simulink model "NEWTstRigidVehicleModelMPC"  (R2023a)
settings: Solver=VariableStepAuto  StartTime=0.0  StopTime=t_step  RelTol=1e-3
values from neighbouring files (symbols this model uses):
  curr_pose = out.Pose.signals.values(end,1:4)    [main2.m]
  g = 9.8    [checkSlip.m]    (also in globalDef.m)
  init_speed = curr_speed    [main2.m]
  M = 900    [globalDef.m]
  pacc = simU(i,1)    [main2.m]
  pdelta = simU(i,2)    [main2.m]
libraries: autolibshared x1
settings Model: Creator=Portelinha  LastModifiedBy=Tiago
settings SolverCC: AlgebraicLoopSolver=TrustRegion
settings DebuggingCC: UnconnectedInputMsg=warning  UnconnectedOutputMsg=warning  UnconnectedLineMsg=warning
settings ModelReferenceCC: EnableRefExpFcnMdlSchedulingChecks=on

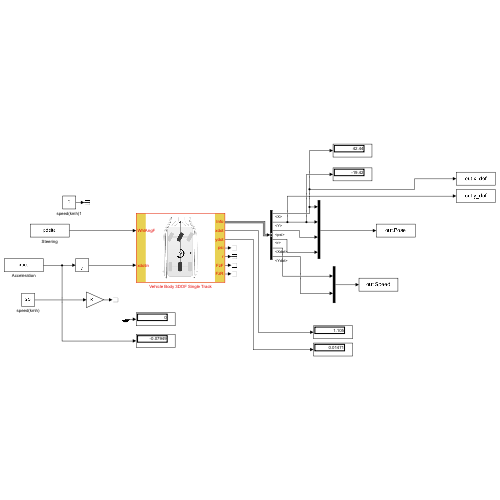
[thumbnail: Simulink's stored preview of the top-level diagram]
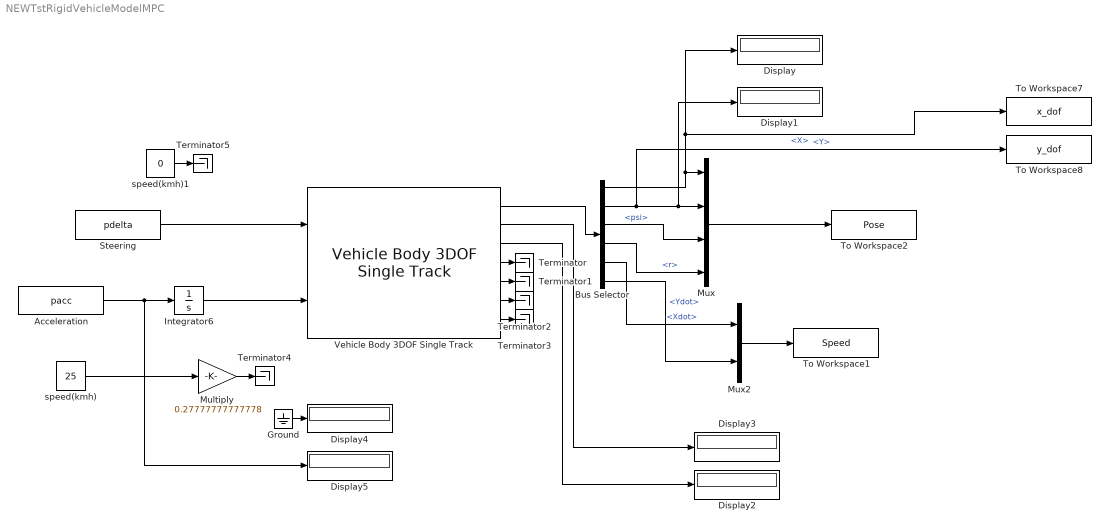
== system NEWTstRigidVehicleModelMPC ==
  Acceleration : Constant  Value=pacc
  Bus Selector : BusSelector  OutputSignals=InertFrm.Cg.Disp.X,InertFrm.Cg.Disp.Y,InertFrm.Cg.Ang.psi,BdyFrm.Cg.AngVel.r,InertFrm.RearAxl.Vel.Xdot,InertFrm.RearAxl.Vel.Ydot
  Display{,1..5} (6 alike) : Display
  Ground : Ground
  Integrator6 : Integrator  InitialCondition=init_speed
  Multiply : Gain  Gain=0.27777777777778
  Mux : Mux
  Mux2 : Mux  Inputs=2
  Steering : Constant  Value=pdelta
  Terminator{,1..5} (6 alike) : Terminator
  To Workspace1 : ToWorkspace  VariableName=Speed  SaveFormat=Structure With Time  SampleTime=-1
  To Workspace2 : ToWorkspace  VariableName=Pose  SaveFormat=Structure With Time  SampleTime=-1
  To Workspace7 : ToWorkspace  VariableName=x_dof  SaveFormat=Structure With Time  SampleTime=-1
  To Workspace8 : ToWorkspace  VariableName=y_dof  SaveFormat=Structure With Time  SampleTime=-1
  Vehicle Body 3DOF Single Track : autolibshared/Vehicle Body 3DOF Single Track  trackMode=Single (bicycle)  inputMode=External longitudinal velocity  frontSteerMode=on  rearSteerMode=off  windMode=off  muMode=off  extFMode=off  extMMode=off  htchFMode=off  htchMMode=off  extXo=off  extpsio=off  extxdoto=off  extro=off  extYo=off  extTamb=off  extydoto=off  aMode=2  NF=2  NR=2  m=900  a=1.25  b=1.25  h=0.35  dh=1  hh=0.2  X_o=curr_pose(1)  xdot_o=0  CalphaMode=off  sigmaMode=on  d=0  hl=0  w=[1.4,1.4]  Cy_f=12e3*5  Cy_r=11e3*5  sigma_f=.1  sigma_r=.1  alpha_f_brk=[-.1 .1]  Cy_f_data=[-9e3 9e3]  alpha_r_brk=[-.1 .1]  Cy_r_data=[-9e3 9e3]  Y_o=curr_pose(2)  ydot_o=vy  Izz=4000  psi_o=curr_pose(3)  r_o=curr_pose(4)  Af=2.14  Cd=0.33  Cl=.1  Cpm=.1  beta_w=[0:0.01:0.3]  Cs=[0:0.03:0.9]  Cym=[0:0.01:0.3]  Pabs=101325  Tair=273  g=9.81  mu=1  xdot_tol=.01  Fznom=M*g  Fxtire_sat=7e4  Fytire_sat=7e4  longOff=0  latOff=0  vertOff=0  wrapAng=off
  speed(kmh) : Constant  Value=25
  speed(kmh)1 : Constant  Value=0
  wires:
  Acceleration/1 -> Display5/1, Integrator6/1
  Vehicle Body 3DOF Single Track/1 -> Bus Selector/1
  Bus Selector/1 -> To Workspace7/1, Display/1, Mux/1  "<X>"
  Bus Selector/2 -> To Workspace8/1, Display1/1, Mux/2  "<Y>"
  Mux/1 -> To Workspace2/1
  Bus Selector/3 -> Mux/3  "<psi>"
  Mux2/1 -> To Workspace1/1
  Bus Selector/4 -> Mux/4  "<r>"
  speed(kmh)/1 -> Multiply/1
  Vehicle Body 3DOF Single Track/2 -> Display3/1
  Vehicle Body 3DOF Single Track/3 -> Display2/1
  Steering/1 -> Vehicle Body 3DOF Single Track/1
  Bus Selector/5 -> Mux2/1  "<Xdot>"
  Bus Selector/6 -> Mux2/2  "<Ydot>"
  Integrator6/1 -> Vehicle Body 3DOF Single Track/2
  Vehicle Body 3DOF Single Track/4 -> Terminator/1
  Vehicle Body 3DOF Single Track/5 -> Terminator1/1
  Vehicle Body 3DOF Single Track/6 -> Terminator2/1
  Vehicle Body 3DOF Single Track/7 -> Terminator3/1
  Multiply/1 -> Terminator4/1
  speed(kmh)1/1 -> Terminator5/1
  Ground/1 -> Display4/1
